simulink model "UAM_Flight_control"  (R2024b)
settings: Solver=FixedStepAuto  StartTime=0.0  StopTime=inf  RelTol=1e-3  EnableMultiTasking=on
undefined symbols (not defined in the file): CityMission, control, controlParams, ControlSampleTime, Cruise_a, DiscIntNeverNeededParam, Earth, FixedWingMission, flightState, FSState, FWControlParams, FWTrimSpeed, HoverMission, params, position, R_WAYPOINTTRANSITION, TransitionMission, uavParam, Vt, w_trim, WGS84, zGround
libraries: slpidlib x56, simulink x35, uavalgslib x8, robotcorelib x2, simulink_extras x2, mspfiltlib x1, aerolibtransform2 x1
(part 12 of 12)

== matlab function UAM_Flight_control/Controller/Auto1/Multicopter Controller/Attitude & Altitude controller/Altitude Control/MATLAB Function2 ==
  data: target_z input; pos_sp output; current_z input; current_vz input; reset input; dt input; vel_ff output; acc_ff output
function [pos_sp, vel_ff, acc_ff] = trajGen(target_z, current_z, current_vz, reset, dt)
    % 좌표계: altitude-up (양수 = 위)

    persistent pos vel acc
    if isempty(pos) || reset
        pos = current_z;
        vel = current_vz;
        acc = 0;
    end

    max_jerk = 4.0;
    max_acc_up = 4.0;
    max_acc_down = 3.0;
    max_vel_up = 3.0;
    max_vel_down = 1.5;

    error = target_z - pos;

    if error > 0
        acc_lim = max_acc_up;
    else
        acc_lim = max_acc_down;
    end

    if vel > 0
        dec_lim = max_acc_down;
    else
        dec_lim = max_acc_up;
    end

    stopping_dist = vel^2 / (2 * dec_lim);

    if (abs(error) > stopping_dist && sign(error) == sign(vel)) || abs(vel) < 0.01
        desired_acc = sign(error) * acc_lim;
    else
        desired_acc = -sign(vel) * dec_lim;
    end

    jerk = (desired_acc - acc) / dt;
    if abs(jerk) > max_jerk
        jerk = sign(jerk) * max_jerk;
    end
    acc = acc + jerk * dt;

    % 이전 속도 저장
    vel_prev = vel;

    % 속도 클램프
    vel_raw = vel + acc * dt;
    vel_clamped = min(max(vel_raw, -max_vel_down), max_vel_up);
    if abs(vel_clamped - vel_raw) > 1e-6
        acc = 0;
    end
    vel = vel_clamped;

    % 사다리꼴 적분
    pos = pos + 0.5 * (vel_prev + vel) * dt;

    if abs(target_z - pos) < 0.01 && abs(vel) < 0.05
        pos = target_z; vel = 0; acc = 0;
    end

    pos_sp = pos;
    vel_ff = vel;
    acc_ff = acc;
end

% ============================================================
% 연결 구조
% ============================================================
%
% HoverSPBus.Z (z_ref) --> [trajGen] --pos_sp--> Position P 입력 (기존 z_ref 자리)
%                                      |--vel_ff--> Position P 출력에 (+) 합산
%                                      |--acc_ff--> Velocity PID 출력에 (+) 합산
%
% trajGen 입력:
%   target_z   <-- HoverSPBus.Z (기존 z_ref)
%   current_z  <-- States.Xe(3) (Gain(-1) 거친 altitude-up)
%   current_vz <-- States.Ve(3) (Gain(-1) 거친 altitude-up)
%   reset      <-- Auto 진입 OR Takeoff 시작 OR target jump > threshold
%   dt         <-- 0.005 (200Hz)
%
% 제어 수식:
%   vz_sp    = P_z * (pos_sp - z) + vel_ff
%   acc_sp_z = PID_vz(vz_sp - vz) + acc_ff
%   acc_sp_z에서 끊고, acc_sp_x/y/z를 모아 thrustToAttitude로 전달
%
% 좌표계:
%   Altitude Control 내부 전체: altitude-up 통일
%   NED 변환은 thrustToAttitude 직전 한 군데에서만 처리
